simulink model "sp1500WECSminiProject"  (R2019b)
settings: Solver=ode8  StartTime=0.0  StopTime=1  FixedStep=0.00001  RelTol=1e-3
values from neighbouring files (symbols this model uses):
  D1 = (Ls*Lr) - (Lm.^2)    [WECSConstants.m]
  Lm = 2.1346*10^(-3)    (= 0.0021346)    [WECSConstants.m]
  Lr = (0.06492*10^(-3)) + (2.1346*10^(-3))    (= 0.00219952)    [WECSConstants.m]
  Ls = (0.06492*10^(-3)) + (2.1346*10^(-3))    (= 0.00219952)    [WECSConstants.m]
  P = 2    [WECSConstants.m]
  Rr = 1.497*10^(-3)    (= 0.001497)    [WECSConstants.m]
  Rs = 1.102*10^(-3)    (= 0.001102)    [WECSConstants.m]
libraries: powerlib x8
settings Model: Creator=Waseem  LastModifiedBy=SONY
settings DataIOCC: LimitDataPoints=on  SaveFormat=Array  SignalLoggingSaveFormat=ModelDataLogs  ReturnWorkspaceOutputs=off
settings OptimizationCC: BlockReduction=off  BooleanDataType=off  LifeSpan=inf
settings DebuggingCC: SaveWithParameterizedLinksMsg=none  UnderspecifiedInitializationDetection=Classic  MergeDetectMultiDrivingBlocksExec=none  SignalResolutionControl=TryResolveAllWithWarning  MultiTaskDSMMsg=warning  MultiTaskCondExecSysMsg=none  StateNameClashWarn=warning  SFUnexpectedBacktrackingDiag=warning  SFNoUnconditionalDefaultTransitionDiag=warning  SFExecutionAtInitializationDiag=none  ArithmeticOperatorsInVariantConditions=warning
settings HardwareCC: ProdBitPerPointer=32  ProdBitPerSizeT=32  ProdBitPerPtrDiffT=32  ProdLargestAtomicFloat=None  ProdIntDivRoundTo=Undefined  ProdEndianess=Unspecified  ProdWordSize=32  ProdHWDeviceType=32-bit Generic  TargetUnknown=on
settings ModelReferenceCC: PropagateSignalLabelsOutOfModel=off
settings SFSimCC: SimUseLocalCustomCode=off  CustomCodeUndefinedFunction=UseInterfaceOnly
settings RTWCC: RTWUseLocalCustomCode=off
settings CodeAppCC: StateflowObjectComments=on
settings GRTTargetCC: TargetLangStandard=C89/C90 (ANSI)  GeneratePreprocessorConditionals=Disable all
settings ConfigComp: CovMetricSettings=dw  CovHtmlReporting=on  CovSaveCumulativeToWorkspaceVar=on  CovSaveSingleToWorkspaceVar=on  CovExternalEMLEnable=off
settings SimscapeCC: SimscapeNormalizeSystem=off

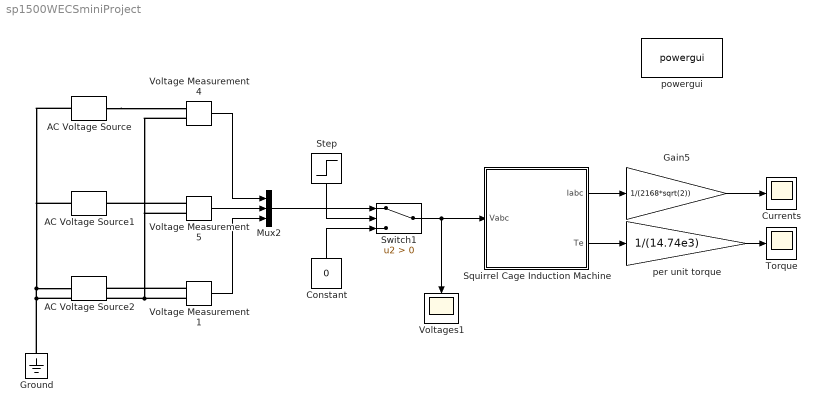
== system sp1500WECSminiProject ==
  AC Voltage Source : powerlib/Electrical Sources/AC Voltage Source  Amplitude=563.38264  Phase=90  Frequency=50  SampleTime=0  Measurements=None  BusType=swing  Pref=10e3  Qref=0  Qmin=-inf  Qmax=+inf
      settings: SourceProductName=Simscape Electrical
  AC Voltage Source1 : powerlib/Electrical Sources/AC Voltage Source  Amplitude=563.38264  Phase=-30  Frequency=50  SampleTime=0  Measurements=None  BusType=swing  Pref=10e3  Qref=0  Qmin=-inf  Qmax=+inf
      settings: SourceProductName=Simscape Electrical
  AC Voltage Source2 : powerlib/Electrical Sources/AC Voltage Source  Amplitude=563.38264  Phase=-150  Frequency=50  SampleTime=0  Measurements=None  BusType=swing  Pref=10e3  Qref=0  Qmin=-inf  Qmax=+inf
      settings: SourceProductName=Simscape Electrical
  Constant : Constant  Value=0
  Currents : Scope
  Gain5 : Gain  Gain=1/(2168*sqrt(2))
  Ground : powerlib/Elements/Ground  LConnTagsString=a
      settings: SourceProductName=Simscape Electrical
  Mux2 : Mux  Inputs=3
  Squirrel Cage Induction Machine : Subsystem
  Step : Step  Time=0.5  SampleTime=0
  Switch1 : Switch  Criteria=u2 > Threshold
  Torque : Scope
  Voltage Measurement1 : powerlib/Measurements/Voltage Measurement  PhasorSimulation=off  OutputType=Complex  PSBequivalent=0
      settings: SourceProductName=Simscape Electrical
  Voltage Measurement4 : powerlib/Measurements/Voltage Measurement  PhasorSimulation=off  OutputType=Complex  PSBequivalent=0
      settings: SourceProductName=Simscape Electrical
  Voltage Measurement5 : powerlib/Measurements/Voltage Measurement  PhasorSimulation=off  OutputType=Complex  PSBequivalent=0
      settings: SourceProductName=Simscape Electrical
  Voltages1 : Scope
  per unit torque : Gain  Gain=1/(14.74e3)
  powergui : powerlib/powergui  Priority=1  SimulationMode=Continuous  SampleTime=50e-6  frequency=50  Iterations=50  frequencyindice=50  Pbase=100e6  ErrMax=1e-4  UnitsV=kV  UnitsW=MW  buscounter=0  FunctionMessages=off  echomessages=off  EnableUseOfTLC=off  CurrentSourceSwitches=on  DisableSnubberDevices=off  DisableRonSwitches=off  DisableVfSwitches=off  DisplayEquations=off  AutomaticDiscreteSolvers=off  SolverType=Tustin  Interpol=off  ExternalGateDelay=off  methode=off  Ts=0  x0status=blocks  SPID=off  SwTol=0  HookPort=off  NonlinearTolerance=1e-4  nMaxIteration=100  ContinueOnMaxIteration=off  RestoreLinks=warning  ResistiveCurrentMeasurement=off  Frange=[0:2:500]  Ylog=off  Xlog=on  ShowGrid=off  save=off  variable=ZData  structure=0  ZoomFFT=off  StartTime=0.0  cycles=1  DisplayStyle=1  fundamental=60  FreqAxis=off  MaxFrequency=1000  frequencyindicesteady=1  RmsSteady=1  display=off
      settings: SourceProductName=Simscape Electrical
  wires:
  Voltage Measurement1/1 -> Mux2/3
  Voltage Measurement5/1 -> Mux2/2
  Squirrel Cage Induction Machine/2(Te) -> per unit torque/1
  Gain5/1 -> Currents/1
  Step/1 -> Switch1/2
  Voltage Measurement4/1 -> Mux2/1
  per unit torque/1 -> Torque/1
  Constant/1 -> Switch1/3
  Switch1/1 -> Voltages1/1, Squirrel Cage Induction Machine/1(Vabc)
  Mux2/1 -> Switch1/1
  Squirrel Cage Induction Machine/1(Iabc) -> Gain5/1
  connections:
  Ground/LConn1 -- AC Voltage Source/LConn1 -- AC Voltage Source1/LConn1 -- AC Voltage Source2/LConn1 -- Voltage Measurement5/LConn2 -- Voltage Measurement4/LConn2 -- Voltage Measurement1/LConn2
  AC Voltage Source/RConn1 -- Voltage Measurement4/LConn1
  Voltage Measurement5/LConn1 -- AC Voltage Source1/RConn1
  Voltage Measurement1/LConn1 -- AC Voltage Source2/RConn1

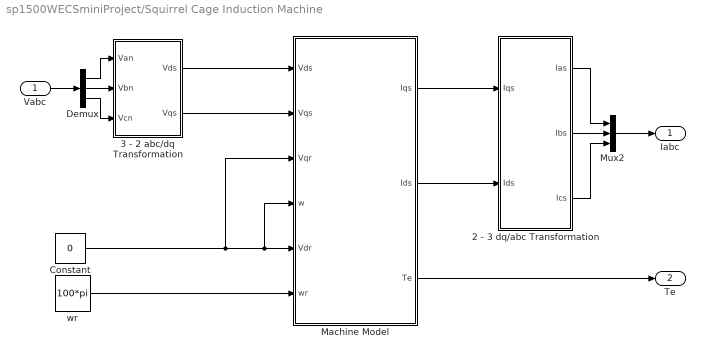
== system sp1500WECSminiProject/Squirrel Cage Induction Machine ==
  Vabc : Inport
  2 - 3 dq/abc Transformation : Subsystem
  3 - 2 abc/dq Transformation : Subsystem
  Constant : Constant  Value=0
  Demux : Demux  Outputs=3
  Machine Model : Subsystem
  Mux2 : Mux  Inputs=3
  wr : Constant  Value=100*pi
  Iabc : Outport
  Te : Outport  Port=2
  wires:
  2 - 3 dq/abc Transformation/2(Ibs) -> Mux2/2
  2 - 3 dq/abc Transformation/3(Ics) -> Mux2/3
  2 - 3 dq/abc Transformation/1(Ias) -> Mux2/1
  Constant/1 -> Machine Model/3(Vqr), Machine Model/4(w), Machine Model/5(Vdr)
  Machine Model/1(Iqs) -> 2 - 3 dq/abc Transformation/1(Iqs)
  3 - 2 abc/dq Transformation/1(Vds) -> Machine Model/1(Vds)
  Machine Model/2(Ids) -> 2 - 3 dq/abc Transformation/2(Ids)
  3 - 2 abc/dq Transformation/2(Vqs) -> Machine Model/2("Vqs ")
  Machine Model/3(Te) -> Te/1
  wr/1 -> Machine Model/6(wr)
  Demux/1 -> 3 - 2 abc/dq Transformation/1(Van)
  Demux/2 -> 3 - 2 abc/dq Transformation/2(Vbn)
  Demux/3 -> 3 - 2 abc/dq Transformation/3(Vcn)
  Vabc/1 -> Demux/1
  Mux2/1 -> Iabc/1

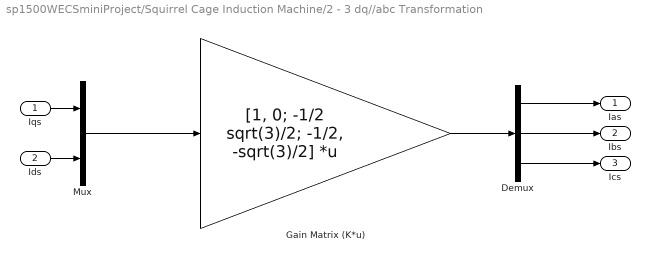
== system sp1500WECSminiProject/Squirrel Cage Induction Machine/2 - 3 dq//abc Transformation ==
  Iqs : Inport
  Ids : Inport  Port=2
  Demux : Demux  Outputs=3
  Gain Matrix (K*u) : Gain  Gain=[1, 0; -1/2 sqrt(3)/2; -1/2, -sqrt(3)/2]  Multiplication=Matrix(K*u)
  Mux : Mux  Inputs=2
  Ias : Outport
  Ibs : Outport  Port=2
  Ics : Outport  Port=3
  wires:
  Mux/1 -> Gain Matrix (K*u)/1
  Gain Matrix (K*u)/1 -> Demux/1
  Demux/2 -> Ibs/1
  Demux/1 -> Ias/1
  Demux/3 -> Ics/1
  Iqs/1 -> Mux/1
  Ids/1 -> Mux/2

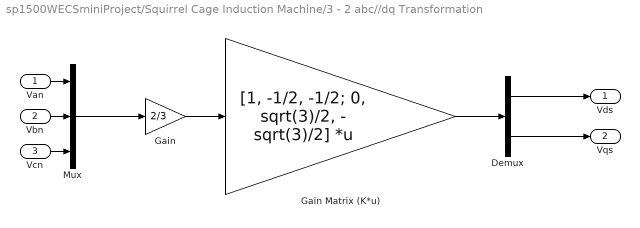
== system sp1500WECSminiProject/Squirrel Cage Induction Machine/3 - 2 abc//dq Transformation ==
  Van : Inport
  Vbn : Inport  Port=2
  Vcn : Inport  Port=3
  Demux : Demux  Outputs=2
  Gain : Gain  Gain=2/3
  Gain Matrix (K*u) : Gain  Gain=[1, -1/2, -1/2; 0, sqrt(3)/2, - sqrt(3)/2]  Multiplication=Matrix(K*u)
  Mux : Mux  Inputs=3
  Vds : Outport
  Vqs : Outport  Port=2
  wires:
  Vcn/1 -> Mux/3
  Vbn/1 -> Mux/2
  Van/1 -> Mux/1
  Gain/1 -> Gain Matrix (K*u)/1
  Gain Matrix (K*u)/1 -> Demux/1
  Mux/1 -> Gain/1
  Demux/1 -> Vds/1
  Demux/2 -> Vqs/1

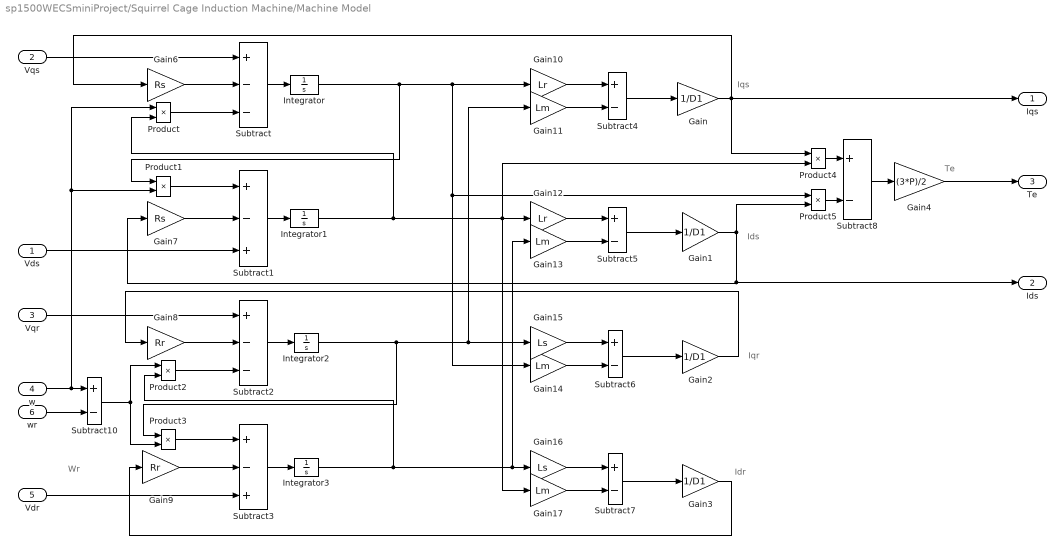
== system sp1500WECSminiProject/Squirrel Cage Induction Machine/Machine Model ==
  note: Idr
  note: Iqr
  note: Te
  note: Ids
  note: Iqs
  note: Wr
  Vds : Inport
  "Vqs " : Inport  Port=2
  Vqr : Inport  Port=3
  w : Inport  Port=4
  Vdr : Inport  Port=5
  wr : Inport  Port=6
  Gain{,1..3} (4 alike) : Gain  Gain=1/D1
  Gain10 : Gain  Gain=Lr
  Gain{11,13..14,17} (4 alike) : Gain  Gain=Lm
  Gain12 : Gain  Gain=Lr
  Gain15 : Gain  Gain=Ls
  Gain16 : Gain  Gain=Ls
  Gain4 : Gain  Gain=(3*P)/2
  Gain6 : Gain  Gain=Rs
  Gain7 : Gain  Gain=Rs
  Gain8 : Gain  Gain=Rr
  Gain9 : Gain  Gain=Rr
  Integrator{,1..3} (4 alike) : Integrator
  Product{,1..5} (6 alike) : Product
  Subtract : Sum  Inputs=+--
  Subtract1 : Sum  Inputs=+-+
  Subtract{4..8,10} (6 alike) : Sum  Inputs=+-
  Subtract2 : Sum  Inputs=+--
  Subtract3 : Sum  Inputs=+-+
  Iqs : Outport
  Ids : Outport  Port=2
  Te : Outport  Port=3
  wires:
  Subtract/1 -> Integrator/1
  Integrator/1 -> Gain10/1, Product5/1, Gain14/1, Product1/1
  Subtract1/1 -> Integrator1/1
  Subtract2/1 -> Integrator2/1
  Subtract3/1 -> Integrator3/1
  Subtract4/1 -> Gain/1
  Subtract5/1 -> Gain1/1
  Subtract6/1 -> Gain2/1
  Subtract7/1 -> Gain3/1
  Subtract8/1 -> Gain4/1
  Product4/1 -> Subtract8/1
  Gain/1 -> Product4/1, Iqs/1, Gain6/1
  Gain10/1 -> Subtract4/1
  Gain11/1 -> Subtract4/2
  Gain6/1 -> Subtract/2
  Product/1 -> Subtract/3
  Product1/1 -> Subtract1/1
  Gain7/1 -> Subtract1/2
  w/1 -> Product/1, Product1/2, Subtract10/1
  Gain12/1 -> Subtract5/1
  Gain13/1 -> Subtract5/2
  Gain1/1 -> Gain7/1, Ids/1, Product5/2
  Product5/1 -> Subtract8/2
  Gain4/1 -> Te/1
  Gain8/1 -> Subtract2/2
  Product2/1 -> Subtract2/3
  Vqr/1 -> Subtract2/1
  Gain14/1 -> Subtract6/2
  Gain15/1 -> Subtract6/1
  Integrator2/1 -> Gain11/1, Gain15/1, Product3/1
  Gain2/1 -> Gain8/1
  Subtract10/1 -> Product3/2, Product2/1
  Product3/1 -> Subtract3/1
  Gain9/1 -> Subtract3/2
  Integrator3/1 -> Gain13/1, Gain16/1, Product2/2
  Gain16/1 -> Subtract7/1
  Gain17/1 -> Subtract7/2
  Gain3/1 -> Gain9/1
  Vdr/1 -> Subtract3/3
  Vds/1 -> Subtract1/3
  "Vqs "/1 -> Subtract/1
  Integrator1/1 -> Gain17/1, Product4/2, Gain12/1, Product/2
  wr/1 -> Subtract10/2
